simulink model "sampleModel1467_3"  (R2023a)
settings: Solver=VariableStepAuto  StartTime=0.0  StopTime=10.0  RelTol=1e-3
libraries: hdlsllib x5, simulink x1
settings Model: Creator=user1  LastModifiedBy=user1

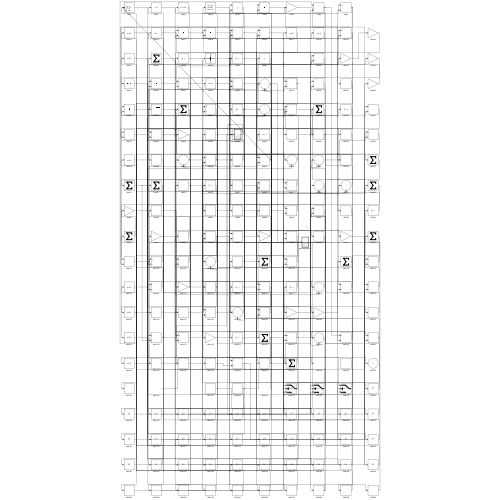
[thumbnail: Simulink's stored preview of the top-level diagram]
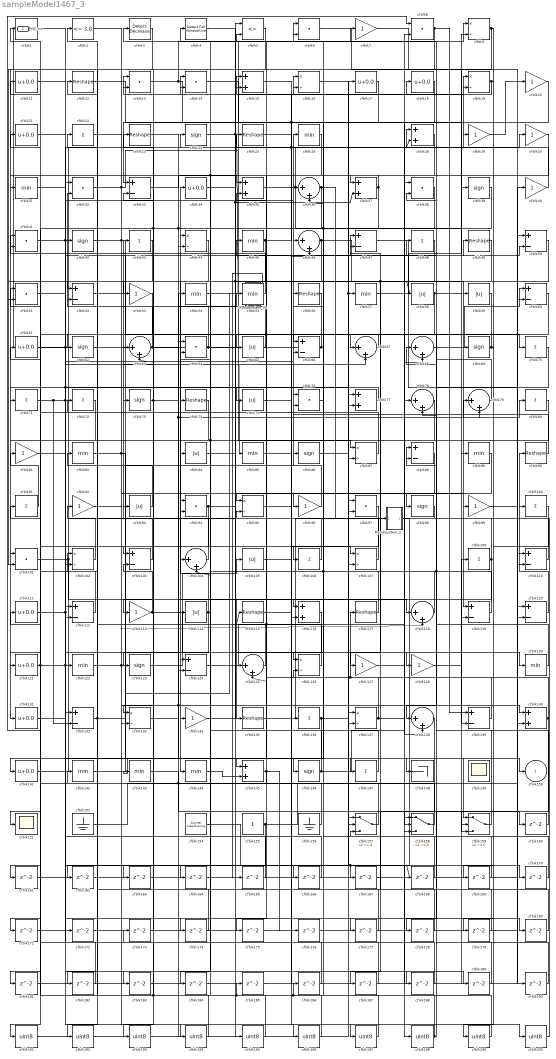
== system sampleModel1467_3 ==
  Mysubsystem_1 : Subsystem  TreatAsAtomicUnit=on  RTWFcnName=Mysubsystem_1
      settings: RTWFcnNameOpts=User specified  RTWFileNameOpts=Use function name
  Mysubsystem_31 : Subsystem  TreatAsAtomicUnit=on  RTWFcnName=Mysubsystem_31
      settings: RTWFcnNameOpts=User specified  RTWFileNameOpts=Use function name
  cfblk1 : hdlsllib/Logic and Bit Operations/Compare To Constant  relop=<=  const=3.0  OutDataTypeStr=uint8
  cfblk{22,43,48,70..72,80,91,100,106,109,136,147} (13 alike) : Sum  Inputs=+  OutDataTypeStr=uint8
  cfblk{6,8,13..14,32,38,41,51,64,76,94,97,101} (13 alike) : DotProduct  OutDataTypeStr=uint8
  cfblk{9,16,19,44,87,95,102,107,126,133,137} (11 alike) : Product  Inputs=*/  OutDataTypeStr=uint8  RndMeth=Zero  SaturateOnIntegerOverflow=on
  cfblk{33,47,50,52,60,66,88,103,110,112,119..120,124,132,139} (15 alike) : Sum  Inputs=+-  OutDataTypeStr=uint8
  cfblk{36,46,63,67..68,78..79,104,118,125,138} (11 alike) : Sum  Inputs=|++  OutDataTypeStr=uint8
  cfblk{58..59,65,75,84,93,105,114} (8 alike) : Abs  OutDataTypeStr=uint8  SaturateOnIntegerOverflow=off
  cfblk{11,17..18,21,34,61,111,121,131,141} (10 alike) : Bias  Bias=0.0  SaturateOnIntegerOverflow=off
  cfblk{7,20,29..30,40,53,81,92,96,99,113,127..128,134} (14 alike) : Gain  OutDataTypeStr=uint8
  cfblk{12,23,25,49,56,74,90,115,117,135} (10 alike) : Reshape
  cfblk{15,28,35,37,77,116,140,145} (8 alike) : Sum  OutDataTypeStr=uint8
  cfblk{26,31,45,54..55,57,82,85,89,122,130,142..144} (14 alike) : MinMax  OutDataTypeStr=uint8
  cfblk{24,39,42,62,69,73,86,98,123,146} (10 alike) : Signum
  cfblk148 : Terminator
  cfblk149 : Scope
      settings: Floating=on
  cfblk151 : Scope
  cfblk152 : Ground
  cfblk154 : hdlsllib/Sources/Counter Free-Running  NumBits=16  tsamp=-1
  cfblk155 : Constant  OutDataTypeStr=uint8  SampleTime=-1
  cfblk156 : Ground
  cfblk157 : Switch  OutDataTypeStr=uint8  SaturateOnIntegerOverflow=off  InputSameDT=off
  cfblk158 : Switch  OutDataTypeStr=uint8  SaturateOnIntegerOverflow=off  InputSameDT=off
  cfblk159 : Switch  OutDataTypeStr=uint8  SaturateOnIntegerOverflow=off  InputSameDT=off
  cfblk{160..190} (31 alike) : Delay  SampleTime=1
  cfblk{191..200} (10 alike) : DataTypeConversion  OutDataTypeStr=uint8  SaturateOnIntegerOverflow=off  RndMeth=Floor
  cfblk2 : hdlsllib/Logic and Bit Operations/Compare To Constant  relop=<=  const=3.0  OutDataTypeStr=uint8
  cfblk3 : simulink/Logic and Bit Operations/Detect Decrease  vinit=0.0  OutDataTypeStr=uint8
      settings: LibrarySourceBlock=|
      | hdlsllib/Logic and Bit
      | Operations/Detect
      | Decrease
  cfblk4 : hdlsllib/Logic and Bit Operations/Detect Fall Nonpositive  vinit=0  OutDataTypeStr=uint8
  cfblk5 : RelationalOperator  Operator=<=  OutDataTypeStr=boolean  InputSameDT=off
  cfblk150 : Outport  OutDataTypeStr=uint8  VectorParamsAs1DForOutWhenUnconnected=off
  Hdl_out : Outport  Port=2  OutDataTypeStr=uint8
  wires:
  cfblk96/1 -> cfblk26/1
  cfblk42/1 -> cfblk70/1, cfblk189/1
  cfblk141/1 -> cfblk24/1
  cfblk25/1 -> cfblk67/1, cfblk28/2
  cfblk142/1 -> cfblk86/1
  cfblk122/1 -> cfblk47/1, cfblk139/2
  cfblk109/1 -> cfblk144/1, cfblk14/2
  cfblk94/1 -> cfblk143/1, cfblk158/2
  cfblk120/1 -> cfblk90/1
  cfblk72/1 -> cfblk131/1
  cfblk114/1 -> cfblk34/1, cfblk133/1
  cfblk29/1 -> cfblk20/1
  cfblk68/1 -> cfblk60/1
  cfblk145/1 -> cfblk175/1, cfblk176/1
  cfblk90/1 -> cfblk76/1
  cfblk32/1 -> cfblk18/1, cfblk118/2
  cfblk119/1 -> cfblk56/1, cfblk13/1, cfblk88/1
  cfblk28/1 -> cfblk37/1
  cfblk48/1 -> cfblk134/1
  cfblk24/1 -> cfblk128/1, cfblk58/1, cfblk85/1
  cfblk104/1 -> cfblk43/1
  cfblk8/1 -> cfblk101/1, cfblk139/1
  cfblk4/1 -> cfblk196/1
  cfblk121/1 -> cfblk8/1, cfblk67/2
  cfblk49/1 -> cfblk96/1
  cfblk112/1 -> cfblk61/1
  cfblk135/1 -> cfblk17/1
  cfblk80/1 -> cfblk112/2, cfblk104/1
  cfblk101/1 -> cfblk135/1, cfblk15/2
  cfblk91/1 -> cfblk81/1
  cfblk123/1 -> cfblk105/1
  cfblk111/1 -> cfblk66/2, cfblk200/1
  cfblk17/1 -> cfblk33/1
  cfblk125/1 -> cfblk22/1
  cfblk35/1 -> cfblk19/1, cfblk69/1
  cfblk113/1 -> cfblk130/1, cfblk103/2
  cfblk64/1 -> cfblk87/1, cfblk42/1
  cfblk154/1 -> cfblk198/1
  cfblk75/1 -> cfblk167/1, cfblk168/1
  cfblk7/1 -> cfblk110/2
  cfblk20/1 -> cfblk137/2
  cfblk157/1 -> cfblk115/1, cfblk15/1
  cfblk137/1 -> cfblk46/1, cfblk79/1
  cfblk106/1 -> cfblk14/1
  cfblk54/1 -> cfblk9/1
  cfblk82/1 -> cfblk159/1, cfblk99/1
  cfblk77/1 -> cfblk71/1
  cfblk126/1 -> cfblk82/1
  cfblk67/1 -> cfblk62/1
  cfblk140/1 -> cfblk73/1, cfblk178/1
  cfblk63/1 -> cfblk32/2, cfblk118/1
  cfblk39/1 -> cfblk116/1, cfblk121/1
  cfblk23/1 -> cfblk148/1, cfblk140/2
  cfblk52/1 -> cfblk77/1
  cfblk139/1 -> cfblk117/1, cfblk44/1
  cfblk87/1 -> cfblk41/1
  cfblk74/1 -> cfblk114/1
  cfblk30/1 -> cfblk104/2, cfblk163/1
  cfblk16/1 -> cfblk57/1, cfblk159/3
  cfblk155/1 -> cfblk40/1, cfblk193/1
  cfblk13/1 -> cfblk136/1, cfblk7/1
  cfblk46/1 -> cfblk119/1, cfblk102/2
  cfblk50/1 -> cfblk127/1, cfblk151/1
  cfblk69/1 -> cfblk66/1, cfblk179/1
  cfblk26/1 -> cfblk145/1
  cfblk156/1 -> cfblk51/1
  cfblk102/1 -> cfblk92/1
  cfblk78/1 -> cfblk84/1
  cfblk134/1 -> cfblk30/1, cfblk37/2
  cfblk132/1 -> Mysubsystem_31/1(In1), cfblk102/1
  cfblk59/1 -> cfblk78/2
  cfblk95/1 -> cfblk49/1
  cfblk45/1 -> cfblk19/2, cfblk51/2
  cfblk60/1 -> cfblk126/1
  cfblk47/1 -> cfblk120/1
  cfblk65/1 -> cfblk23/1
  cfblk40/1 -> cfblk25/1
  cfblk85/1 -> cfblk107/1
  cfblk124/1 -> cfblk38/1
  cfblk55/1 -> cfblk21/1
  cfblk73/1 -> cfblk98/1, cfblk79/2, cfblk103/1
  cfblk118/1 -> cfblk93/1, cfblk6/2
  cfblk158/1 -> cfblk142/1
  cfblk159/1 -> cfblk94/1
  cfblk144/1 -> cfblk145/2
  cfblk41/1 -> cfblk5/1, cfblk36/1
  cfblk81/1 -> cfblk48/1
  cfblk2/1 -> cfblk194/1
  cfblk6/1 -> cfblk39/1
  cfblk37/1 -> cfblk31/1, cfblk184/1
  cfblk147/1 -> cfblk64/2
  cfblk56/1 -> cfblk123/1
  cfblk58/1 -> cfblk113/1, cfblk125/2, cfblk140/1
  cfblk133/1 -> cfblk55/1
  cfblk110/1 -> cfblk74/1
  cfblk18/1 -> cfblk146/1
  cfblk70/1 -> cfblk138/1
  cfblk36/1 -> Mysubsystem_1/1(In1), cfblk63/2, cfblk133/2, cfblk44/2
  cfblk79/1 -> cfblk45/1
  cfblk146/1 -> cfblk29/1, cfblk5/2
  cfblk89/1 -> cfblk95/1
  cfblk31/1 -> cfblk122/1, cfblk183/1
  cfblk66/1 -> cfblk65/1, Hdl_out/1
  cfblk1/1 -> cfblk124/1, cfblk77/2
  cfblk130/1 -> cfblk3/1
  cfblk5/1 -> cfblk53/1
  cfblk76/1 -> cfblk6/1
  cfblk152/1 -> cfblk8/2, cfblk124/2
  cfblk43/1 -> cfblk52/1
  cfblk57/1 -> cfblk9/2
  cfblk88/1 -> cfblk106/1
  cfblk93/1 -> cfblk72/1
  cfblk14/1 -> cfblk138/2
  cfblk127/1 -> cfblk68/2
  cfblk71/1 -> cfblk28/1, cfblk164/1, cfblk132/2
  cfblk19/1 -> cfblk13/2, cfblk169/1
  cfblk107/1 -> cfblk16/1
  cfblk100/1 -> cfblk199/1
  cfblk12/1 -> cfblk116/2, cfblk89/1
  cfblk128/1 -> cfblk109/1
  cfblk115/1 -> cfblk147/1
  cfblk84/1 -> cfblk80/1
  cfblk116/1 -> cfblk125/1
  cfblk86/1 -> cfblk157/2
  cfblk38/1 -> cfblk141/1
  cfblk103/1 -> cfblk12/1
  cfblk136/1 -> cfblk170/1, cfblk171/1
  cfblk33/1 -> cfblk35/1
  cfblk9/1 -> cfblk59/1, cfblk101/2
  cfblk61/1 -> cfblk150/1, cfblk50/2
  cfblk98/1 -> cfblk95/2
  cfblk22/1 -> cfblk75/1
  cfblk117/1 -> cfblk35/2
  cfblk143/1 -> cfblk160/1
  cfblk160/1 -> cfblk126/2
  cfblk53/1 -> cfblk161/1
  cfblk161/1 -> cfblk158/1
  cfblk162/1 -> cfblk107/2
  cfblk163/1 -> cfblk60/2
  cfblk164/1 -> cfblk87/2
  cfblk165/1 -> cfblk132/1
  cfblk92/1 -> cfblk166/1
  cfblk166/1 -> cfblk63/1
  cfblk167/1 -> cfblk78/1
  cfblk168/1 -> cfblk36/2
  cfblk169/1 -> cfblk157/1
  cfblk170/1 -> cfblk47/2
  cfblk171/1 -> cfblk119/2
  cfblk11/1 -> cfblk172/1
  cfblk172/1 -> cfblk110/1
  cfblk173/1 -> cfblk33/2
  cfblk21/1 -> cfblk174/1
  cfblk174/1 -> cfblk52/2
  cfblk175/1 -> cfblk137/1
  cfblk176/1 -> cfblk120/2
  cfblk51/1 -> cfblk177/1
  cfblk177/1 -> cfblk94/2
  cfblk178/1 -> cfblk157/3
  cfblk179/1 -> cfblk16/2
  cfblk15/1 -> cfblk180/1
  cfblk180/1 -> cfblk64/1
  cfblk44/1 -> cfblk181/1
  cfblk181/1 -> cfblk50/1
  cfblk62/1 -> cfblk182/1
  cfblk182/1 -> cfblk41/2
  cfblk183/1 -> cfblk46/2
  cfblk184/1 -> cfblk159/2
  cfblk185/1 -> cfblk158/3
  cfblk186/1 -> cfblk1/1
  cfblk138/1 -> cfblk187/1
  cfblk187/1 -> cfblk112/1
  cfblk131/1 -> cfblk188/1
  cfblk188/1 -> cfblk32/1
  cfblk189/1 -> cfblk38/2
  cfblk99/1 -> cfblk190/1
  cfblk190/1 -> cfblk68/1
  cfblk97/1 -> cfblk191/1
  cfblk191/1 -> cfblk54/1
  cfblk3/1 -> cfblk192/1
  cfblk192/1 -> cfblk97/1
  cfblk193/1 -> cfblk97/2
  cfblk194/1 -> cfblk173/1, cfblk11/1
  cfblk34/1 -> cfblk195/1
  cfblk195/1 -> cfblk2/1
  cfblk196/1 -> cfblk186/1, cfblk111/1
  cfblk105/1 -> cfblk197/1
  cfblk197/1 -> cfblk4/1
  cfblk198/1 -> cfblk88/2, cfblk76/2
  cfblk199/1 -> cfblk185/1, cfblk91/1
  cfblk200/1 -> cfblk100/1
  Mysubsystem_1/1(Out1) -> cfblk162/1
  Mysubsystem_31/1(Out1) -> cfblk165/1

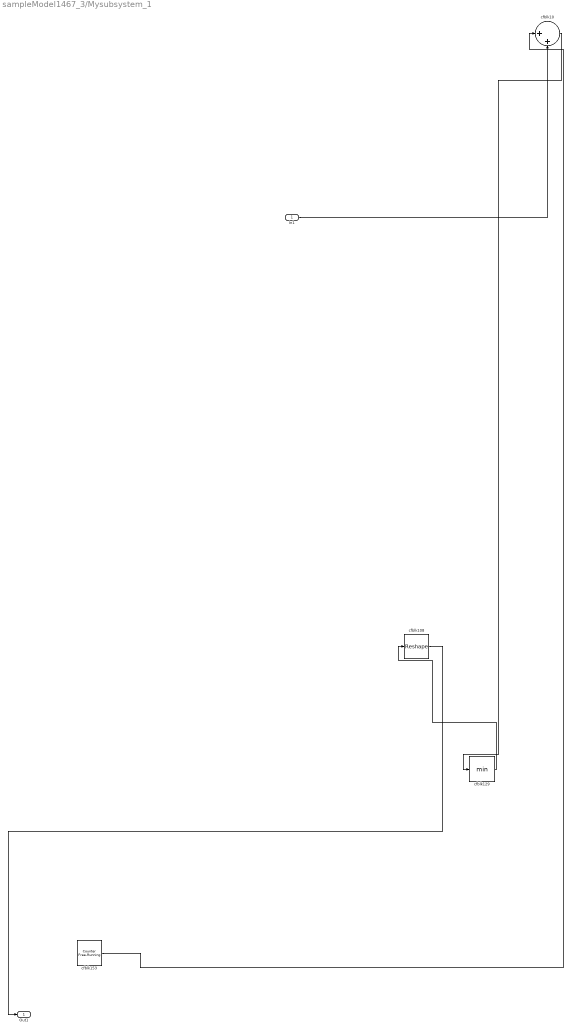
== system sampleModel1467_3/Mysubsystem_1 ==
  In1 : Inport
  cfblk10 : Sum  Inputs=|++
  cfblk108 : Reshape
  cfblk129 : MinMax
  cfblk153 : hdlsllib/Sources/Counter Free-Running  NumBits=16  tsamp=-1
  Out1 : Outport
  wires:
  cfblk153/1 -> cfblk10/1
  cfblk10/1 -> cfblk129/1
  cfblk108/1 -> Out1/1
  cfblk129/1 -> cfblk108/1
  In1/1 -> cfblk10/2

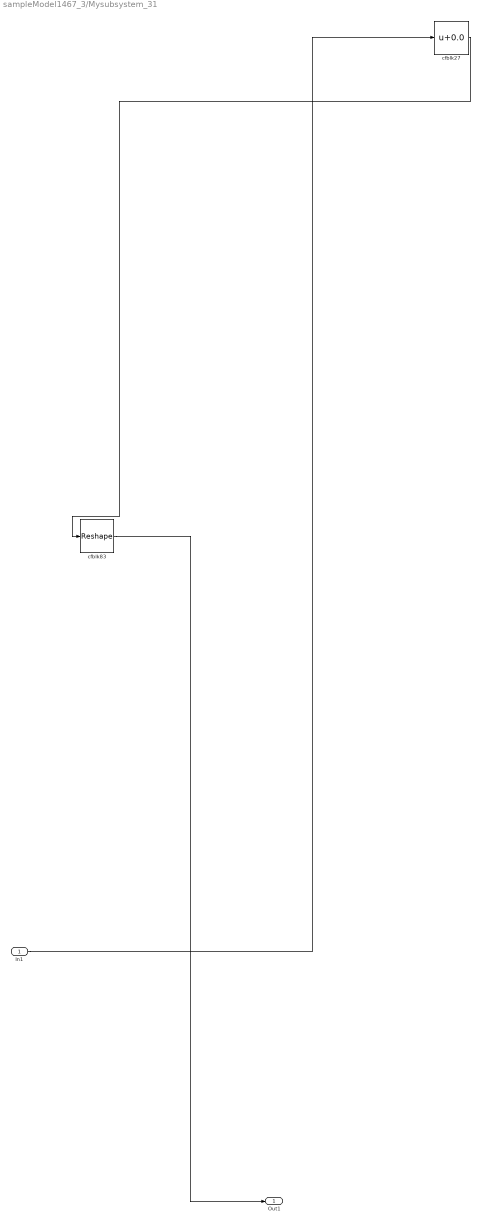
== system sampleModel1467_3/Mysubsystem_31 ==
  In1 : Inport
  cfblk27 : Bias  Bias=0.0  SaturateOnIntegerOverflow=off
  cfblk83 : Reshape
  Out1 : Outport
  wires:
  cfblk83/1 -> Out1/1
  cfblk27/1 -> cfblk83/1
  In1/1 -> cfblk27/1
